simulink model "untitled"  (R2024b)
settings: Solver=VariableStepAuto  StartTime=0.0  StopTime=10.0  RelTol=1e-3
settings Model: Creator=DT User  LastModifiedBy=DT User

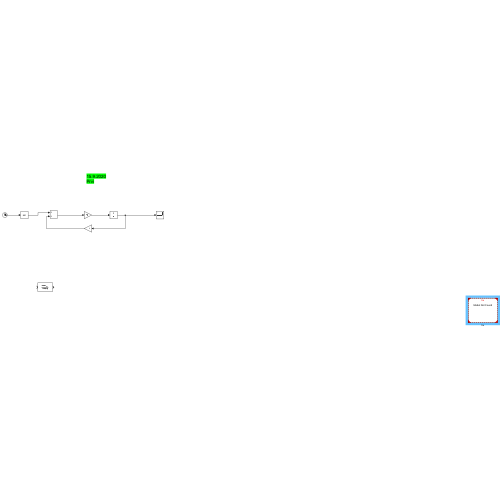
[thumbnail: Simulink's stored preview of the top-level diagram]
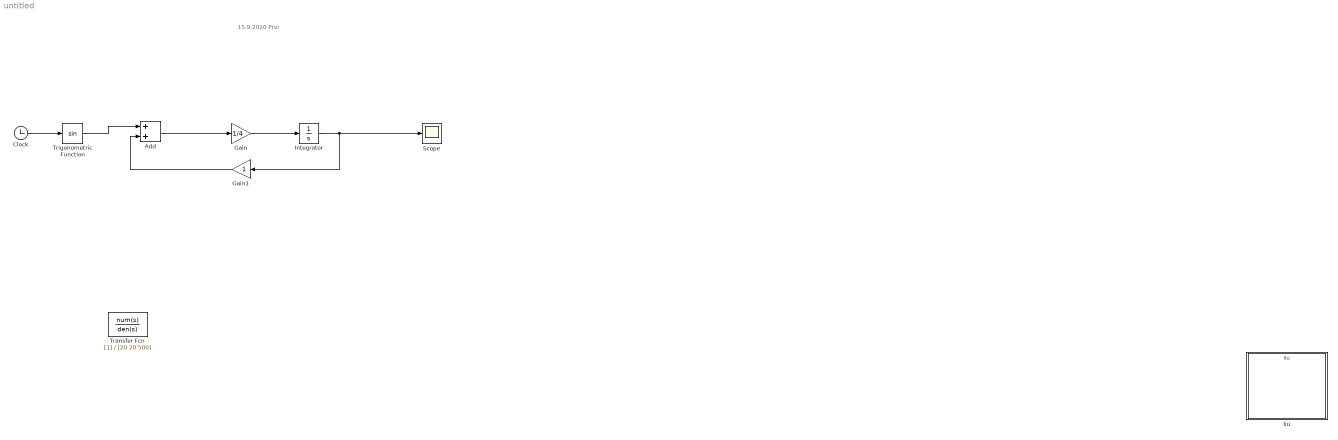
== system untitled ==
  note: 15.9.2020
      | Prvi
  Add : Sum
  Clock : Clock
  Gain : Gain  Gain=1/4
  Gain1 : Gain
  Integrator : Integrator
  Scope : Scope
  Transfer Fcn : TransferFcn  Denominator=[20 20 500]
  Trigonometric Function : Trigonometry
  liu : ModelReference  ModelNameDialog=liu.slx  SimulationMode=Normal
  wires:
  Gain/1 -> Integrator/1
  Integrator/1 -> Gain1/1, Scope/1
  Clock/1 -> Trigonometric Function/1
  Trigonometric Function/1 -> Add/1
  Add/1 -> Gain/1
  Gain1/1 -> Add/2
